simulink model "transimpedance_amplifier_TSV620AILT"  (R2024a)
settings: Solver=VariableStepAuto  StartTime=0.0  StopTime=10.0  RelTol=1e-3
undefined symbols (not defined in the file): x, y
libraries: fl_lib x46, nesl_utility x22, simulink x4, ee_lib x2
settings Model: Creator=timot  LastModifiedBy=timot

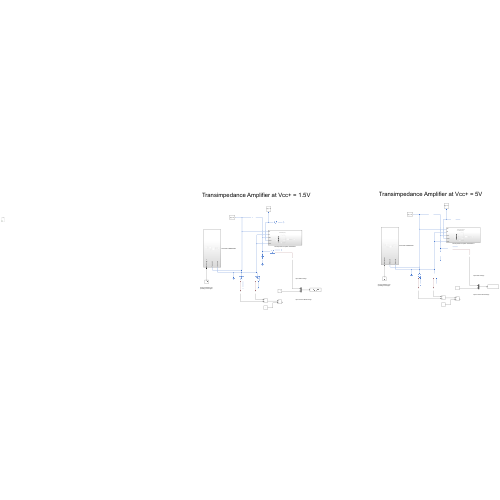
[thumbnail: Simulink's stored preview of the top-level diagram]
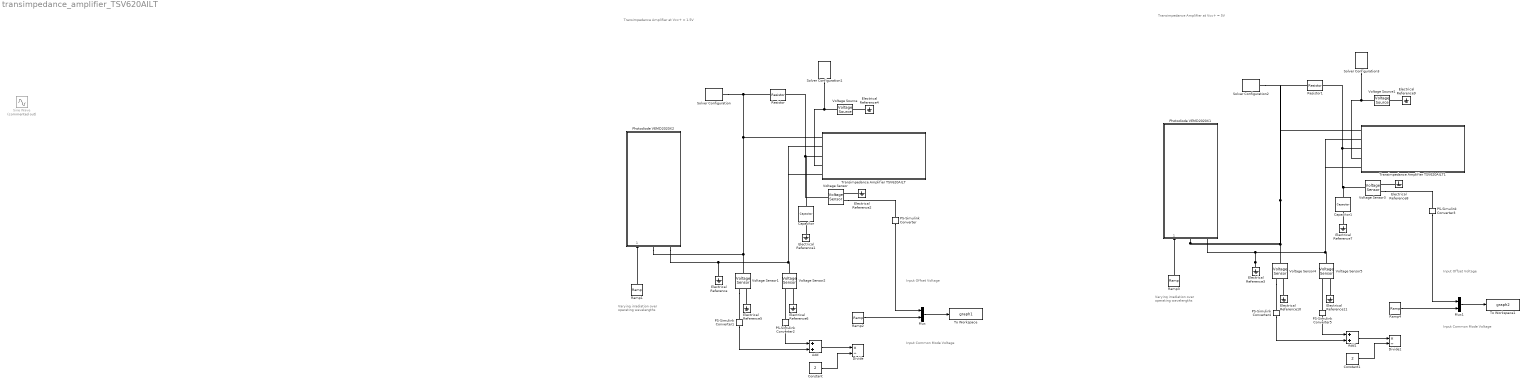
== system transimpedance_amplifier_TSV620AILT ==
  note: Transimpedance Amplifier at Vcc+ = 5V
  note: Varying irradiation over
      | operating wavelengths
  note: Input Common Mode Voltage
  note: Input Offset Voltage
  note: Input Common Mode Voltage
  note: Varying irradiation over
      | operating wavelengths
  note: Input Offset Voltage
  note: Transimpedance Amplifier at Vcc+ = 1.5V
  Add : Sum
  Add1 : Sum
  Capacitor : fl_lib/Electrical/Electrical Elements/Capacitor  c=100 nF  r=1e-6 Ohm  g=0 1/Ohm  i_specify=off  i_priority=None  i=0 A  i_nominal_specify=off  i_nominal_value=1  i_nominal_unit=A  v_specify=off  v_priority=None  v=0 V  v_nominal_specify=off  v_nominal_value=1  v_nominal_unit=V  vc_specify=off  vc_priority=High  vc=0 V  vc_nominal_specify=off  vc_nominal_value=1  vc_nominal_unit=V
  Capacitor1 : fl_lib/Electrical/Electrical Elements/Capacitor  c=100 nF  r=1e-6 Ohm  g=0 1/Ohm  i_specify=off  i_priority=None  i=0 A  i_nominal_specify=off  i_nominal_value=1  i_nominal_unit=A  v_specify=off  v_priority=None  v=0 V  v_nominal_specify=off  v_nominal_value=1  v_nominal_unit=V  vc_specify=off  vc_priority=High  vc=0 V  vc_nominal_specify=off  vc_nominal_value=1  vc_nominal_unit=V
  Constant : Constant  Value=2
  Constant1 : Constant  Value=2
  Divide : Product  Inputs=*/
  Divide1 : Product  Inputs=*/
  Electrical Reference{,1..11} (12 alike) : fl_lib/Electrical/Electrical Elements/Electrical Reference
  Mux : Mux  Inputs=2
  Mux1 : Mux  Inputs=2
  PS-Simulink Converter{,1..5} (6 alike) : nesl_utility/PS-Simulink Converter  PhysicalDomain=network_engine_domain  SubClassName=ps_output  LeftPortType=input  RightPortType=output  PseudoPeriodic=off  Frequencies=[]  VectorFormat=inherit  Unit=inherit  AffineConversion=off
  Photodiode VEMD2020X1 : Subsystem
  Photodiode VEMD2020X2 : Subsystem
  Ramp1 : simulink/Sources/Ramp  slope=1e-8  start=0  InitialOutput=8.5e-7
  Ramp2 : simulink/Sources/Ramp  slope=0.19  start=0  InitialOutput=-0.2
  Ramp3 : simulink/Sources/Ramp  slope=1e-8  start=0  InitialOutput=8.5e-7
  Ramp4 : simulink/Sources/Ramp  slope=0.19  start=0  InitialOutput=-0.2
  Resistor : fl_lib/Electrical/Electrical Elements/Resistor  R=127 kOhm  i_specify=off  i_priority=None  i=0 A  i_nominal_specify=off  i_nominal_value=1  i_nominal_unit=A  v_specify=off  v_priority=None  v=0 V  v_nominal_specify=off  v_nominal_value=1  v_nominal_unit=V
  Resistor1 : fl_lib/Electrical/Electrical Elements/Resistor  R=127 kOhm  i_specify=off  i_priority=None  i=0 A  i_nominal_specify=off  i_nominal_value=1  i_nominal_unit=A  v_specify=off  v_priority=None  v=0 V  v_nominal_specify=off  v_nominal_value=1  v_nominal_unit=V
  Sine Wave : Sin  Commented=on  SampleTime=0
  Solver Configuration{,1..3} (4 alike) : nesl_utility/Solver Configuration  PhysicalDomain=network_engine_domain  SubClassName=solver  LeftPortType=input  RightPortType=generic  Tones=[]  Harmonics=[]  SimulateNoise=off  Profile=off  UseLocalSampling=off  EnableSwitchedLinearOptims=on  FrequencyDomain=off  UseCCode=off  RelTol=0.001  AbsTol=0.001  MinStep=1e-09  ToWorkspace=off  RevertToSquareIcSolve=off  NumHomotopyIterations=100  PhasorMode=off  PhasorModeNumHarmonics=1  ConsistencySolver=NEWTON_XTOL_AFTER_FTOL  IndexReductionMethod=DerivativeReplacement  DoDC=off  ResidualTolerance=1e-09  ConsistencyTolSource=GLOBAL  ConsistencyAbsTol=0.001  ConsistencyRelTol=0.001  ConsistencyTolFactor=0.001  UseLocalSolver=off  LocalSolverChoice=NE_BACKWARD_EULER_ADVANCER  ResolveIndetEquations=on  FunctionEvalNumThread=1  LocalSolverSampleTime=0.001  DoFixedCost=off  MaxNonlinIter=3  MaxModeIter=2  ComputeImpulses=off  ImpulseIterations=2  LinearAlgebra=auto  LinearAlgebraNumThread=0  EquationFormulation=NE_TIME_EF  DelaysMemoryBudget=1024  AutomaticFiltering=on  FilteringTimeConstant=0.001  PartitionStorageMethod=AS_NEEDED  PartitionMemoryBudget=1024  PartitionMethod=ROBUST  MultibodyUseLocalSolver=off  MultibodyLocalSolverChoice=ODE1  MultibodyLocalSolverSampleTime=0.001
  To Workspace : ToWorkspace  VariableName=graph1  SaveFormat=Timeseries  SampleTime=-1
  To Workspace1 : ToWorkspace  VariableName=graph2  SaveFormat=Timeseries  SampleTime=-1
  Transimpedance Amplifier TSV620AILT : Subsystem
  Transimpedance Amplifier TSV620AILT1 : Subsystem
  Voltage Sensor{,1..5} (6 alike) : fl_lib/Electrical/Electrical Sensors/Voltage Sensor
  Voltage Source : ee_lib/Sources/Voltage Source  dc_voltage=1.5 V  ac_voltage=0 V  ac_shift=0 rad  ac_frequency=60 Hz  noise_mode=ee.enum.sources.noise.Disabled  PSD=0 V^2/Hz  sample_time=1e-3 s  repeatability=ee.enum.sources.repeatability.NotRepeatable  user_seed=0  auto_seed=3499211588  i_specify=off  i_priority=None  i=0 A  i_nominal_specify=off  i_nominal_value=1  i_nominal_unit=A  v_specify=off  v_priority=None  v=0 V  v_nominal_specify=off  v_nominal_value=1  v_nominal_unit=V
  Voltage Source1 : ee_lib/Sources/Voltage Source  dc_voltage=5 V  ac_voltage=0 V  ac_shift=0 rad  ac_frequency=60 Hz  noise_mode=ee.enum.sources.noise.Disabled  PSD=0 V^2/Hz  sample_time=1e-3 s  repeatability=ee.enum.sources.repeatability.NotRepeatable  user_seed=0  auto_seed=545404223  i_specify=off  i_priority=None  i=0 A  i_nominal_specify=off  i_nominal_value=1  i_nominal_unit=A  v_specify=off  v_priority=None  v=0 V  v_nominal_specify=off  v_nominal_value=1  v_nominal_unit=V
  wires:
  PS-Simulink Converter2/1 -> Add/1
  PS-Simulink Converter1/1 -> Add/2
  Add/1 -> Divide/1
  Constant/1 -> Divide/2
  Mux/1 -> To Workspace/1
  PS-Simulink Converter/1 -> Mux/1
  Ramp1/1 -> Photodiode VEMD2020X2/1("Wavelength, λ")
  Ramp2/1 -> Mux/2
  Mux1/1 -> To Workspace1/1
  PS-Simulink Converter3/1 -> Mux1/1
  Constant1/1 -> Divide1/2
  Ramp4/1 -> Mux1/2
  PS-Simulink Converter4/1 -> Add1/2
  Ramp3/1 -> Photodiode VEMD2020X1/1("Wavelength, λ")
  Add1/1 -> Divide1/1
  PS-Simulink Converter5/1 -> Add1/1
  connections:
  Transimpedance Amplifier TSV620AILT/LConn2 -- Transimpedance Amplifier TSV620AILT/LConn5 -- Voltage Sensor2/LConn1 -- Photodiode VEMD2020X2/LConn2 -- Electrical Reference/LConn1
  Transimpedance Amplifier TSV620AILT/LConn1 -- Solver Configuration/RConn1 -- Resistor/LConn1 -- Photodiode VEMD2020X2/LConn1 -- Voltage Sensor1/LConn1
  Transimpedance Amplifier TSV620AILT/LConn3 -- Voltage Sensor/LConn1 -- Capacitor/LConn1 -- Resistor/RConn1
  Electrical Reference1/LConn1 -- Capacitor/RConn1
  Electrical Reference2/LConn1 -- Voltage Sensor/RConn2
  Voltage Sensor/RConn1 -- PS-Simulink Converter/LConn1
  Solver Configuration1/RConn1 -- Voltage Source/LConn1 -- Transimpedance Amplifier TSV620AILT/LConn4
  Electrical Reference4/LConn1 -- Voltage Source/RConn1
  Electrical Reference5/LConn1 -- Voltage Sensor1/RConn2
  Voltage Sensor1/RConn1 -- PS-Simulink Converter1/LConn1
  Electrical Reference6/LConn1 -- Voltage Sensor2/RConn2
  PS-Simulink Converter2/LConn1 -- Voltage Sensor2/RConn1
  Solver Configuration3/RConn1 -- Transimpedance Amplifier TSV620AILT1/LConn4 -- Voltage Source1/LConn1
  Capacitor1/LConn1 -- Resistor1/RConn1 -- Transimpedance Amplifier TSV620AILT1/LConn3 -- Voltage Sensor3/LConn1
  Electrical Reference3/LConn1 -- Transimpedance Amplifier TSV620AILT1/LConn2 -- Transimpedance Amplifier TSV620AILT1/LConn5 -- Voltage Sensor5/LConn1 -- Photodiode VEMD2020X1/LConn2
  Photodiode VEMD2020X1/LConn1 -- Voltage Sensor4/LConn1 -- Solver Configuration2/RConn1 -- Resistor1/LConn1 -- Transimpedance Amplifier TSV620AILT1/LConn1
  PS-Simulink Converter5/LConn1 -- Voltage Sensor5/RConn1
  Electrical Reference9/LConn1 -- Voltage Source1/RConn1
  Electrical Reference10/LConn1 -- Voltage Sensor4/RConn2
  Electrical Reference11/LConn1 -- Voltage Sensor5/RConn2
  Voltage Sensor4/RConn1 -- PS-Simulink Converter4/LConn1
  Electrical Reference8/LConn1 -- Voltage Sensor3/RConn2
  Electrical Reference7/LConn1 -- Capacitor1/RConn1
  Voltage Sensor3/RConn1 -- PS-Simulink Converter3/LConn1

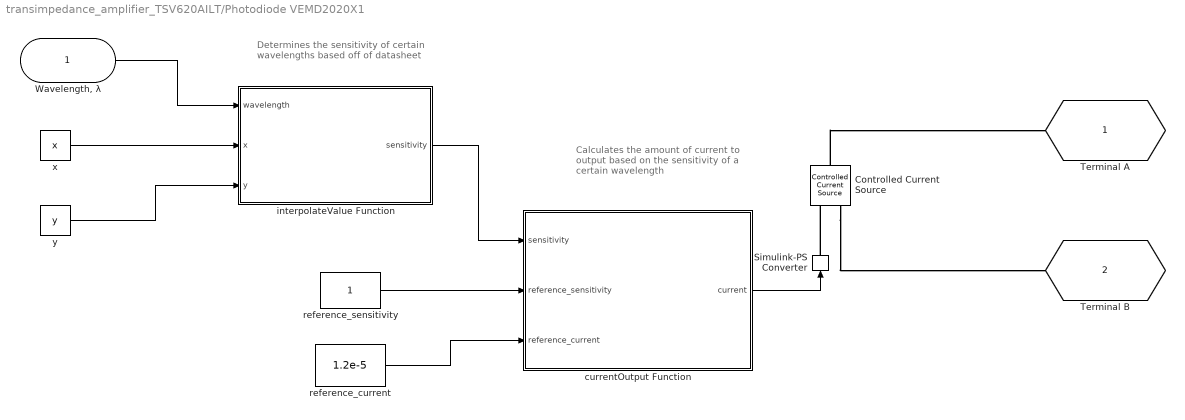
== system transimpedance_amplifier_TSV620AILT/Photodiode VEMD2020X1 ==
  note: Determines the sensitivity of certain
      | wavelengths based off of datasheet
  note: Calculates the amount of current
      | to output based on the sensitivity
      | of a certain wavelength
  "Wavelength, λ" : Inport
  Controlled Current Source : fl_lib/Electrical/Electrical Sources/Controlled Current Source
  Simulink-PS Converter : nesl_utility/Simulink-PS Converter  PhysicalDomain=network_engine_domain  SubClassName=ps_input  LeftPortType=input  RightPortType=output  PseudoPeriodic=off  Frequencies=[]  NoiseDistribution=none  NoiseParameters=[]  Unit=1  AffineConversion=off  FilteringAndDerivatives=provide  SimscapeFilterOrder=1  InputFilterTimeConstant=0.001  UdotUserProvided=0
  currentOutput Function : MATLAB Function  TreatAsAtomicUnit=on
  interpolateValue Function : MATLAB Function  TreatAsAtomicUnit=on
  reference_current : Constant  Value=1.2e-5
  reference_sensitivity : Constant
  x : Constant  Value=x
  y : Constant  Value=y
  Terminal A : PMIOPort  Side=Left
  Terminal B : PMIOPort  Port=2  Side=Left
  wires:
  interpolateValue Function/1(sensitivity) -> currentOutput Function/1(sensitivity)
  x/1 -> interpolateValue Function/2(x)
  currentOutput Function/1(current) -> Simulink-PS Converter/1
  reference_sensitivity/1 -> currentOutput Function/2(reference_sensitivity)
  reference_current/1 -> currentOutput Function/3(reference_current)
  "Wavelength, λ"/1 -> interpolateValue Function/1(wavelength)
  y/1 -> interpolateValue Function/3(y)
  connections:
  Simulink-PS Converter/RConn1 -- Controlled Current Source/RConn1
  Controlled Current Source/RConn2 -- Terminal B/RConn1
  Controlled Current Source/LConn1 -- Terminal A/RConn1

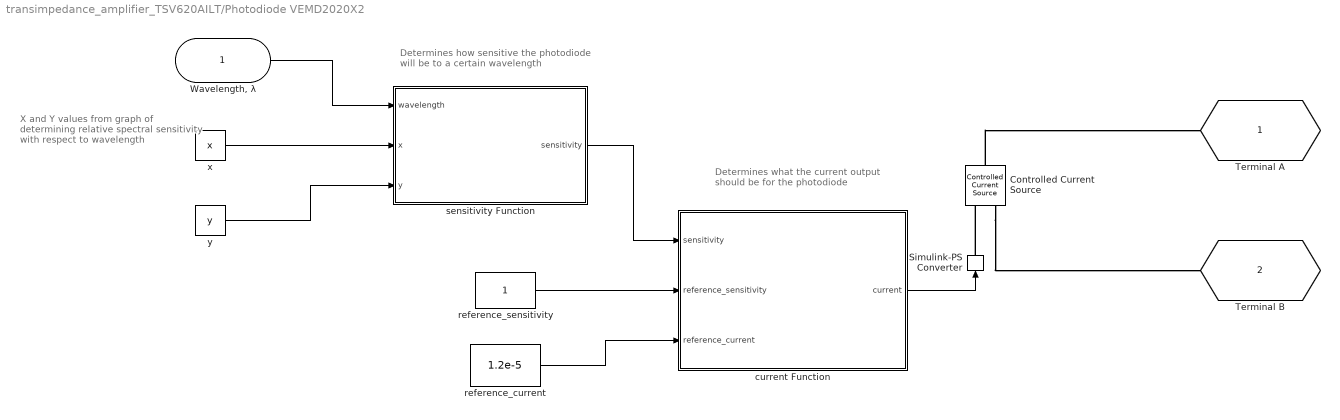
== system transimpedance_amplifier_TSV620AILT/Photodiode VEMD2020X2 ==
  note: Determines what the current
      | output should be for the photodiode
  note: Determines how sensitive the photodiode
      | will be to a certain wavelength
  note: X and Y values from graph of
      | determining relative spectral
      | sensitivity with respect to wavelength
  "Wavelength, λ" : Inport
  Controlled Current Source : fl_lib/Electrical/Electrical Sources/Controlled Current Source
  Simulink-PS Converter : nesl_utility/Simulink-PS Converter  PhysicalDomain=network_engine_domain  SubClassName=ps_input  LeftPortType=input  RightPortType=output  PseudoPeriodic=off  Frequencies=[]  NoiseDistribution=none  NoiseParameters=[]  Unit=1  AffineConversion=off  FilteringAndDerivatives=provide  SimscapeFilterOrder=1  InputFilterTimeConstant=0.001  UdotUserProvided=0
  current Function : MATLAB Function  TreatAsAtomicUnit=on
  reference_current : Constant  Value=1.2e-5
  reference_sensitivity : Constant
  sensitivity Function : MATLAB Function  TreatAsAtomicUnit=on
  x : Constant  Value=x
  y : Constant  Value=y
  Terminal A : PMIOPort  Side=Left
  Terminal B : PMIOPort  Port=2  Side=Left
  wires:
  sensitivity Function/1(sensitivity) -> current Function/1(sensitivity)
  x/1 -> sensitivity Function/2(x)
  current Function/1(current) -> Simulink-PS Converter/1
  reference_sensitivity/1 -> current Function/2(reference_sensitivity)
  reference_current/1 -> current Function/3(reference_current)
  y/1 -> sensitivity Function/3(y)
  "Wavelength, λ"/1 -> sensitivity Function/1(wavelength)
  connections:
  Simulink-PS Converter/RConn1 -- Controlled Current Source/RConn1
  Controlled Current Source/RConn2 -- Terminal B/RConn1
  Controlled Current Source/LConn1 -- Terminal A/RConn1

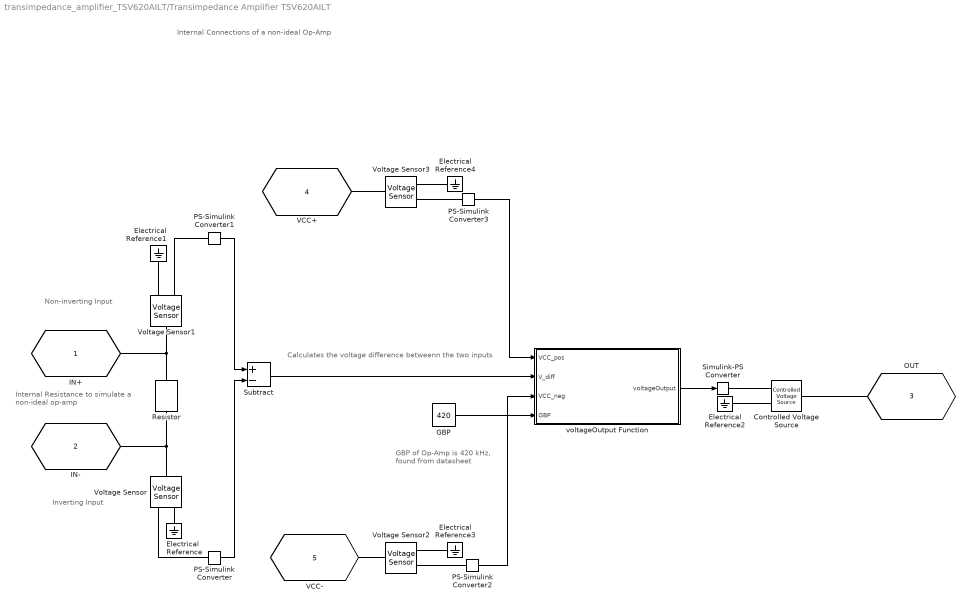
== system transimpedance_amplifier_TSV620AILT/Transimpedance Amplifier TSV620AILT ==
  note: Calculates the voltage difference betweenn the two inputs
  note: Internal Connections of a non-ideal Op-Amp
  note: Internal Resistance to simulate
      | a non-ideal op-amp
  note: Inverting Input
  note: Non-inverting Input
  note: GBP of Op-Amp is 420 kHz,
      | found from datasheet
  Controlled Voltage Source : fl_lib/Electrical/Electrical Sources/Controlled Voltage Source
  Electrical Reference{,1..4} (5 alike) : fl_lib/Electrical/Electrical Elements/Electrical Reference
  GBP : Constant  Value=420
  PS-Simulink Converter{,1..3} (4 alike) : nesl_utility/PS-Simulink Converter  PhysicalDomain=network_engine_domain  SubClassName=ps_output  LeftPortType=input  RightPortType=output  PseudoPeriodic=off  Frequencies=[]  VectorFormat=inherit  Unit=inherit  AffineConversion=off
  Resistor : fl_lib/Electrical/Electrical Elements/Resistor  R=1 GOhm  i_specify=off  i_priority=None  i=0 A  i_nominal_specify=off  i_nominal_value=1  i_nominal_unit=A  v_specify=off  v_priority=None  v=0 V  v_nominal_specify=off  v_nominal_value=1  v_nominal_unit=V
  Simulink-PS Converter : nesl_utility/Simulink-PS Converter  PhysicalDomain=network_engine_domain  SubClassName=ps_input  LeftPortType=input  RightPortType=output  PseudoPeriodic=off  Frequencies=[]  NoiseDistribution=none  NoiseParameters=[]  Unit=1  AffineConversion=off  FilteringAndDerivatives=provide  SimscapeFilterOrder=1  InputFilterTimeConstant=0.001  UdotUserProvided=0
  Subtract : Sum  Inputs=+-
  Voltage Sensor{,1..3} (4 alike) : fl_lib/Electrical/Electrical Sensors/Voltage Sensor
  voltageOutput Function : MATLAB Function  TreatAsAtomicUnit=on
  IN+ : PMIOPort  Side=Left
  IN- : PMIOPort  Port=2  Side=Left
  OUT : PMIOPort  Port=3  Side=Left
  VCC+ : PMIOPort  Port=4  Side=Left
  VCC- : PMIOPort  Port=5  Side=Left
  wires:
  PS-Simulink Converter1/1 -> Subtract/1
  PS-Simulink Converter/1 -> Subtract/2
  voltageOutput Function/1(voltageOutput) -> Simulink-PS Converter/1
  Subtract/1 -> voltageOutput Function/2(V_diff)
  PS-Simulink Converter2/1 -> voltageOutput Function/3(VCC_neg)
  PS-Simulink Converter3/1 -> voltageOutput Function/1(VCC_pos)
  GBP/1 -> voltageOutput Function/4(GBP)
  connections:
  IN+/RConn1 -- Voltage Sensor1/LConn1 -- Resistor/LConn1
  Resistor/RConn1 -- Voltage Sensor/LConn1 -- IN-/RConn1
  Electrical Reference/LConn1 -- Voltage Sensor/RConn2
  Voltage Sensor/RConn1 -- PS-Simulink Converter/LConn1
  Electrical Reference1/LConn1 -- Voltage Sensor1/RConn2
  Voltage Sensor1/RConn1 -- PS-Simulink Converter1/LConn1
  Simulink-PS Converter/RConn1 -- Controlled Voltage Source/RConn1
  Controlled Voltage Source/LConn1 -- OUT/RConn1
  Electrical Reference2/LConn1 -- Controlled Voltage Source/RConn2
  Voltage Sensor2/LConn1 -- VCC-/RConn1
  Electrical Reference3/LConn1 -- Voltage Sensor2/RConn2
  Voltage Sensor2/RConn1 -- PS-Simulink Converter2/LConn1
  Electrical Reference4/LConn1 -- Voltage Sensor3/RConn2
  Voltage Sensor3/RConn1 -- PS-Simulink Converter3/LConn1
  Voltage Sensor3/LConn1 -- VCC+/RConn1

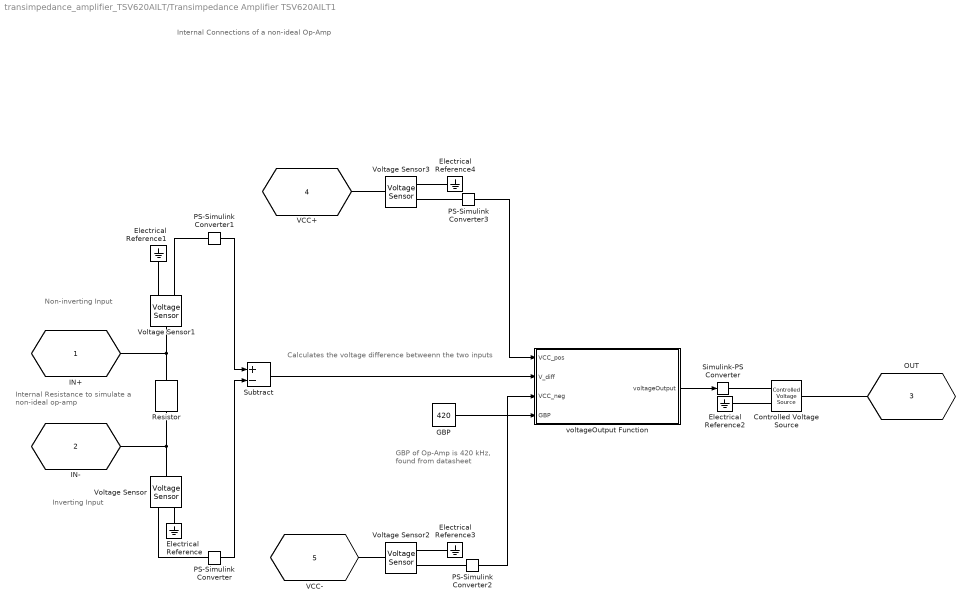
== system transimpedance_amplifier_TSV620AILT/Transimpedance Amplifier TSV620AILT1 ==
  note: Calculates the voltage difference betweenn the two inputs
  note: Internal Connections of a non-ideal Op-Amp
  note: Internal Resistance to simulate
      | a non-ideal op-amp
  note: Inverting Input
  note: Non-inverting Input
  note: GBP of Op-Amp is 420 kHz,
      | found from datasheet
  Controlled Voltage Source : fl_lib/Electrical/Electrical Sources/Controlled Voltage Source
  Electrical Reference{,1..4} (5 alike) : fl_lib/Electrical/Electrical Elements/Electrical Reference
  GBP : Constant  Value=420
  PS-Simulink Converter{,1..3} (4 alike) : nesl_utility/PS-Simulink Converter  PhysicalDomain=network_engine_domain  SubClassName=ps_output  LeftPortType=input  RightPortType=output  PseudoPeriodic=off  Frequencies=[]  VectorFormat=inherit  Unit=inherit  AffineConversion=off
  Resistor : fl_lib/Electrical/Electrical Elements/Resistor  R=1 GOhm  i_specify=off  i_priority=None  i=0 A  i_nominal_specify=off  i_nominal_value=1  i_nominal_unit=A  v_specify=off  v_priority=None  v=0 V  v_nominal_specify=off  v_nominal_value=1  v_nominal_unit=V
  Simulink-PS Converter : nesl_utility/Simulink-PS Converter  PhysicalDomain=network_engine_domain  SubClassName=ps_input  LeftPortType=input  RightPortType=output  PseudoPeriodic=off  Frequencies=[]  NoiseDistribution=none  NoiseParameters=[]  Unit=1  AffineConversion=off  FilteringAndDerivatives=provide  SimscapeFilterOrder=1  InputFilterTimeConstant=0.001  UdotUserProvided=0
  Subtract : Sum  Inputs=+-
  Voltage Sensor{,1..3} (4 alike) : fl_lib/Electrical/Electrical Sensors/Voltage Sensor
  voltageOutput Function : MATLAB Function  TreatAsAtomicUnit=on
  IN+ : PMIOPort  Side=Left
  IN- : PMIOPort  Port=2  Side=Left
  OUT : PMIOPort  Port=3  Side=Left
  VCC+ : PMIOPort  Port=4  Side=Left
  VCC- : PMIOPort  Port=5  Side=Left
  wires:
  PS-Simulink Converter1/1 -> Subtract/1
  PS-Simulink Converter/1 -> Subtract/2
  voltageOutput Function/1(voltageOutput) -> Simulink-PS Converter/1
  Subtract/1 -> voltageOutput Function/2(V_diff)
  PS-Simulink Converter2/1 -> voltageOutput Function/3(VCC_neg)
  PS-Simulink Converter3/1 -> voltageOutput Function/1(VCC_pos)
  GBP/1 -> voltageOutput Function/4(GBP)
  connections:
  IN+/RConn1 -- Voltage Sensor1/LConn1 -- Resistor/LConn1
  Resistor/RConn1 -- Voltage Sensor/LConn1 -- IN-/RConn1
  Electrical Reference/LConn1 -- Voltage Sensor/RConn2
  Voltage Sensor/RConn1 -- PS-Simulink Converter/LConn1
  Electrical Reference1/LConn1 -- Voltage Sensor1/RConn2
  Voltage Sensor1/RConn1 -- PS-Simulink Converter1/LConn1
  Simulink-PS Converter/RConn1 -- Controlled Voltage Source/RConn1
  Controlled Voltage Source/LConn1 -- OUT/RConn1
  Electrical Reference2/LConn1 -- Controlled Voltage Source/RConn2
  Voltage Sensor2/LConn1 -- VCC-/RConn1
  Electrical Reference3/LConn1 -- Voltage Sensor2/RConn2
  Voltage Sensor2/RConn1 -- PS-Simulink Converter2/LConn1
  Electrical Reference4/LConn1 -- Voltage Sensor3/RConn2
  Voltage Sensor3/RConn1 -- PS-Simulink Converter3/LConn1
  Voltage Sensor3/LConn1 -- VCC+/RConn1

== matlab function transimpedance_amplifier_TSV620AILT/Transimpedance Amplifier TSV620AILT/voltageOutput Function ==
  data: VCC_pos input; voltageOutput output; V_diff input; VCC_neg input; GBP input
function voltageOutput = voltageOutput(VCC_pos , V_diff, VCC_neg , GBP)

%Frequency used should be the maximum frequency of the photodiode
rise_time = 1e-7;
max_frequency = 1 / (2*pi*rise_time);
max_frequency = max_frequency / 1000;

%Calculating gain of the Op-Amp
gain = GBP / max_frequency;

voltageOutput = V_diff * gain;

%Ensures the output voltage is within the range of the supply voltages
if voltageOutput < VCC_neg
    voltageOutput = VCC_neg;
elseif voltageOutput > VCC_pos
    voltageOutput = VCC_pos;
end

== matlab function transimpedance_amplifier_TSV620AILT/Photodiode VEMD2020X1/currentOutput Function ==
  data: sensitivity input; current output; reference_sensitivity input; reference_current input
function current = currentOutput(sensitivity, reference_sensitivity, reference_current)

current = reference_current * (sensitivity/reference_sensitivity);

== matlab function transimpedance_amplifier_TSV620AILT/Photodiode VEMD2020X1/interpolateValue Function ==
  data: wavelength input; sensitivity output; x input; y input
function sensitivity = interpolateValue(wavelength, x, y)

if wavelength < 8.3e-7
    error("Invalid wavelength");
elseif wavelength > 9.5e-7
    error("Invalid wavelength");
end

persistent interpFunc;
if isempty(interpFunc)
    interpFunc = @(xq) interp1(x, y, xq, 'linear');
end

sensitivity = interpFunc(wavelength);
end

== matlab function transimpedance_amplifier_TSV620AILT/Transimpedance Amplifier TSV620AILT1/voltageOutput Function ==
  data: VCC_pos input; voltageOutput output; V_diff input; VCC_neg input; GBP input
function voltageOutput = voltageOutput(VCC_pos , V_diff, VCC_neg , GBP)

%Frequency used should be the maximum frequency of the photodiode
rise_time = 1e-7;
max_frequency = 1 / (2*pi*rise_time);
max_frequency = max_frequency / 1000;

%Calculating gain of the Op-Amp
gain = GBP / max_frequency;

voltageOutput = V_diff * gain;

%Ensures the output voltage is within the range of the supply voltages
if voltageOutput < VCC_neg
    voltageOutput = VCC_neg;
elseif voltageOutput > VCC_pos
    voltageOutput = VCC_pos;
end

== matlab function transimpedance_amplifier_TSV620AILT/Photodiode VEMD2020X2/current Function ==
  data: sensitivity input; current output; reference_sensitivity input; reference_current input
function current = current(sensitivity, reference_sensitivity, reference_current)

%Determines current based on sensitivity of the photodiode to a wavelength

current = reference_current * (sensitivity/reference_sensitivity);

== matlab function transimpedance_amplifier_TSV620AILT/Photodiode VEMD2020X2/sensitivity Function ==
  data: wavelength input; sensitivity output; x input; y input
function sensitivity = sensitivity(wavelength, x, y)

%Ensures wavelength is within operational range for photodiode
if wavelength < 8.3e-7
    error("Invalid wavelength");
elseif wavelength > 9.5e-7
    error("Invalid wavelength");
end

%Interpolates the sensitivtiy based on graph from datasheet
persistent interpFunc;
if isempty(interpFunc)
    interpFunc = @(xq) interp1(x, y, xq, 'linear');
end

sensitivity = interpFunc(wavelength);
end
